simulink model "gm_HilbertTransformer"  (R2022a)
settings: Solver=FixedStepDiscrete  StartTime=0.0  StopTime=10.0  RelTol=1e-3
undefined symbols (not defined in the file or in its folder): h_fi
settings Model: Creator=user  LastModifiedBy=user
settings OptimizationCC: BlockReduction=off  ConditionallyExecuteInputs=off  DefaultParameterBehavior=Inlined  InheritOutputTypeSmallerThanSingle=on
settings DebuggingCC: AlgebraicLoopMsg=error  InheritedTsInSrcMsg=none  SingleTaskRateTransMsg=error
settings HardwareCC: ProdBitPerPointer=32  ProdBitPerSizeT=32  ProdBitPerPtrDiffT=32  ProdLargestAtomicFloat=None  ProdIntDivRoundTo=Undefined  ProdEndianess=Unspecified  ProdWordSize=32  ProdHWDeviceType=ASIC/FPGA->ASIC/FPGA  TargetBitPerPointer=64  TargetBitPerSizeT=64  TargetBitPerPtrDiffT=64  TargetLongLongMode=on  TargetIntDivRoundTo=Zero  TargetEndianess=LittleEndian  TargetWordSize=64  TargetHWDeviceType=Custom Processor->MATLAB Host Computer  ProdEqTarget=off

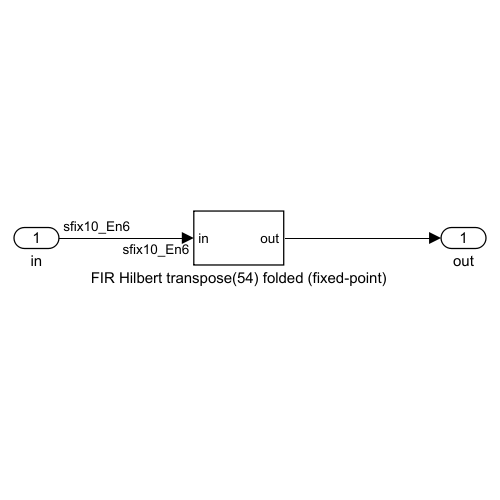
[thumbnail: Simulink's stored preview of the top-level diagram]
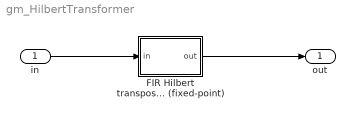
== system gm_HilbertTransformer ==
  in : Inport  OutDataTypeStr=fixdt(1, 10, 6)  PortDimensions=1  SampleTime=0.2
  FIR Hilbert transpose(54) folded (fixed-point) : Subsystem
  out : Outport  SampleTime=0.2
  wires:
  in/1 -> FIR Hilbert transpose(54) folded (fixed-point)/1(in)
  FIR Hilbert transpose(54) folded (fixed-point)/1(out) -> out/1

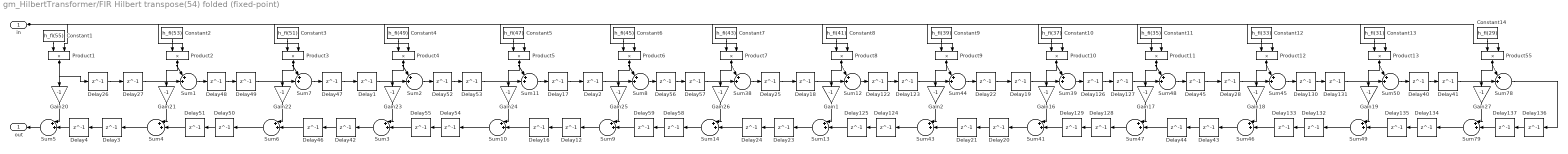
== system gm_HilbertTransformer/FIR Hilbert transpose(54) folded (fixed-point) ==
  in : Inport  OutDataTypeStr=fixdt(1, 10, 6)  PortDimensions=1  SampleTime=0.2
  Constant1 : Constant  Value=h_fi(55)  SampleTime=-1  LockScale=on
  Constant10 : Constant  Value=h_fi(37)  SampleTime=-1  LockScale=on
  Constant11 : Constant  Value=h_fi(35)  SampleTime=-1  LockScale=on
  Constant12 : Constant  Value=h_fi(33)  SampleTime=-1  LockScale=on
  Constant13 : Constant  Value=h_fi(31)  SampleTime=-1  LockScale=on
  Constant14 : Constant  Value=h_fi(29)  SampleTime=-1  LockScale=on
  Constant2 : Constant  Value=h_fi(53)  SampleTime=-1  LockScale=on
  Constant3 : Constant  Value=h_fi(51)  SampleTime=-1  LockScale=on
  Constant4 : Constant  Value=h_fi(49)  SampleTime=-1  LockScale=on
  Constant5 : Constant  Value=h_fi(47)  SampleTime=-1  LockScale=on
  Constant6 : Constant  Value=h_fi(45)  SampleTime=-1  LockScale=on
  Constant7 : Constant  Value=h_fi(43)  SampleTime=-1  LockScale=on
  Constant8 : Constant  Value=h_fi(41)  SampleTime=-1  LockScale=on
  Constant9 : Constant  Value=h_fi(39)  SampleTime=-1  LockScale=on
  Delay{1..4,12,16..28,40..59,122..137} (54 alike) : Delay  DelayLength=1
  Gain{1..2,16,22..26} (8 alike) : Gain  Gain=-1  OutDataTypeStr=fixdt(1,12,12)  RndMeth=Convergent
  Gain17 : Gain  Gain=-1  OutDataTypeStr=fixdt(1,12,11)  RndMeth=Convergent
  Gain18 : Gain  Gain=-1  OutDataTypeStr=fixdt(1,12,11)  RndMeth=Convergent
  Gain19 : Gain  Gain=-1  OutDataTypeStr=fixdt(1,12,10)  RndMeth=Convergent
  Gain20 : Gain  Gain=-1  OutDataTypeStr=fixdt(1,9,9)  RndMeth=Convergent
  Gain21 : Gain  Gain=-1  OutDataTypeStr=fixdt(1,11,11)  RndMeth=Convergent
  Gain27 : Gain  Gain=-1  OutDataTypeStr=fixdt(1,12,8)  RndMeth=Convergent
  Product1 : Product  OutDataTypeStr=fixdt(1,9,9)  RndMeth=Convergent
  Product{3..10} (8 alike) : Product  OutDataTypeStr=fixdt(1,12,12)  RndMeth=Convergent
  Product11 : Product  OutDataTypeStr=fixdt(1,12,11)  RndMeth=Convergent
  Product12 : Product  OutDataTypeStr=fixdt(1,12,11)  RndMeth=Convergent
  Product13 : Product  OutDataTypeStr=fixdt(1,12,10)  RndMeth=Convergent
  Product2 : Product  OutDataTypeStr=fixdt(1,11,11)  RndMeth=Convergent
  Product55 : Product  OutDataTypeStr=fixdt(1,12,8)  RndMeth=Convergent
  Sum{1..2,8,11} (4 alike) : Sum  Inputs=|++||  OutDataTypeStr=fixdt(1,11,11)  RndMeth=Convergent
  Sum{10,46..47,49,78..79} (6 alike) : Sum  Inputs=|++||  OutDataTypeStr=fixdt(1,16,11)  RndMeth=Convergent
  Sum12 : Sum  Inputs=|++||  OutDataTypeStr=fixdt(1,13,12)  RndMeth=Convergent
  Sum{3..6,9,13..14,41,43} (9 alike) : Sum  Inputs=|++||  OutDataTypeStr=fixdt(1,17,12)  RndMeth=Convergent
  Sum38 : Sum  Inputs=|++||  OutDataTypeStr=fixdt(1,13,12)  RndMeth=Convergent
  Sum39 : Sum  Inputs=|++||  OutDataTypeStr=fixdt(1,13,11)  RndMeth=Convergent
  Sum44 : Sum  Inputs=|++||  OutDataTypeStr=fixdt(1,14,12)  RndMeth=Convergent
  Sum45 : Sum  Inputs=|++||  OutDataTypeStr=fixdt(1,14,11)  RndMeth=Convergent
  Sum48 : Sum  Inputs=|++||  OutDataTypeStr=fixdt(1,12,10)  RndMeth=Convergent
  Sum50 : Sum  Inputs=|++||  OutDataTypeStr=fixdt(1,14,11)  RndMeth=Convergent
  Sum7 : Sum  Inputs=|++||  OutDataTypeStr=fixdt(1,12,12)  RndMeth=Convergent
  out : Outport  SampleTime=0.2
  wires:
  in/1 -> Product9/2, Product8/2, Product7/2, Product6/2, Product55/2, Product5/2, Product4/2, Product3/2, Product2/2, Product13/2, Product12/2, Product11/2, Product10/2, Product1/2
  Constant1/1 -> Product1/1
  Constant10/1 -> Product10/1
  Constant11/1 -> Product11/1
  Constant12/1 -> Product12/1
  Constant13/1 -> Product13/1
  Constant14/1 -> Product55/1
  Constant2/1 -> Product2/1
  Constant3/1 -> Product3/1
  Constant4/1 -> Product4/1
  Constant5/1 -> Product5/1
  Constant6/1 -> Product6/1
  Constant7/1 -> Product7/1
  Constant8/1 -> Product8/1
  Constant9/1 -> Product9/1
  Delay1/1 -> Sum2/2
  Delay12/1 -> Delay16/1
  Delay122/1 -> Delay123/1
  Delay123/1 -> Sum44/2
  Delay124/1 -> Delay125/1
  Delay125/1 -> Sum13/2
  Delay126/1 -> Delay127/1
  Delay127/1 -> Sum48/2
  Delay128/1 -> Delay129/1
  Delay129/1 -> Sum41/2
  Delay130/1 -> Delay131/1
  Delay131/1 -> Sum50/2
  Delay132/1 -> Delay133/1
  Delay133/1 -> Sum46/2
  Delay134/1 -> Delay135/1
  Delay135/1 -> Sum49/2
  Delay136/1 -> Delay137/1
  Delay137/1 -> Sum79/2
  Delay16/1 -> Sum10/2
  Delay17/1 -> Delay2/1
  Delay18/1 -> Sum12/2
  Delay19/1 -> Sum39/2
  Delay2/1 -> Sum8/2
  Delay20/1 -> Delay21/1
  Delay21/1 -> Sum43/2
  Delay22/1 -> Delay19/1
  Delay23/1 -> Delay24/1
  Delay24/1 -> Sum14/2
  Delay25/1 -> Delay18/1
  Delay26/1 -> Delay27/1
  Delay27/1 -> Sum1/2
  Delay28/1 -> Sum45/2
  Delay3/1 -> Delay4/1
  Delay4/1 -> Sum5/2
  Delay40/1 -> Delay41/1
  Delay41/1 -> Sum78/2
  Delay42/1 -> Delay46/1
  Delay43/1 -> Delay44/1
  Delay44/1 -> Sum47/2
  Delay45/1 -> Delay28/1
  Delay46/1 -> Sum6/2
  Delay47/1 -> Delay1/1
  Delay48/1 -> Delay49/1
  Delay49/1 -> Sum7/2
  Delay50/1 -> Delay51/1
  Delay51/1 -> Sum4/2
  Delay52/1 -> Delay53/1
  Delay53/1 -> Sum11/2
  Delay54/1 -> Delay55/1
  Delay55/1 -> Sum3/2
  Delay56/1 -> Delay57/1
  Delay57/1 -> Sum38/2
  Delay58/1 -> Delay59/1
  Delay59/1 -> Sum9/2
  Gain1/1 -> Sum13/1
  Gain16/1 -> Sum41/1
  Gain17/1 -> Sum47/1
  Gain18/1 -> Sum46/1
  Gain19/1 -> Sum49/1
  Gain2/1 -> Sum43/1
  Gain20/1 -> Sum5/1
  Gain21/1 -> Sum4/1
  Gain22/1 -> Sum6/1
  Gain23/1 -> Sum3/1
  Gain24/1 -> Sum10/1
  Gain25/1 -> Sum9/1
  Gain26/1 -> Sum14/1
  Gain27/1 -> Sum79/1
  Product1/1 -> Gain20/1, Delay26/1
  Product10/1 -> Sum39/1, Gain16/1
  Product11/1 -> Sum48/1, Gain17/1
  Product12/1 -> Sum45/1, Gain18/1
  Product13/1 -> Sum50/1, Gain19/1
  Product2/1 -> Sum1/1, Gain21/1
  Product3/1 -> Sum7/1, Gain22/1
  Product4/1 -> Sum2/1, Gain23/1
  Product5/1 -> Sum11/1, Gain24/1
  Product55/1 -> Sum78/1, Gain27/1
  Product6/1 -> Sum8/1, Gain25/1
  Product7/1 -> Sum38/1, Gain26/1
  Product8/1 -> Sum12/1, Gain1/1
  Product9/1 -> Sum44/1, Gain2/1
  Sum1/1 -> Delay48/1
  Sum10/1 -> Delay54/1
  Sum11/1 -> Delay17/1
  Sum12/1 -> Delay122/1
  Sum13/1 -> Delay23/1
  Sum14/1 -> Delay58/1
  Sum2/1 -> Delay52/1
  Sum3/1 -> Delay42/1
  Sum38/1 -> Delay25/1
  Sum39/1 -> Delay126/1
  Sum4/1 -> Delay3/1
  Sum41/1 -> Delay20/1
  Sum43/1 -> Delay124/1
  Sum44/1 -> Delay22/1
  Sum45/1 -> Delay130/1
  Sum46/1 -> Delay43/1
  Sum47/1 -> Delay128/1
  Sum48/1 -> Delay45/1
  Sum49/1 -> Delay132/1
  Sum5/1 -> out/1
  Sum50/1 -> Delay40/1
  Sum6/1 -> Delay50/1
  Sum7/1 -> Delay47/1
  Sum78/1 -> Delay136/1
  Sum79/1 -> Delay134/1
  Sum8/1 -> Delay56/1
  Sum9/1 -> Delay12/1
